simulink model "control2_feedback_linearization"  (R2023b)
settings: Solver=VariableStepAuto  StartTime=0.0  StopTime=20  RelTol=1e-3
values from neighbouring files (symbols this model uses):
  d = obs_r+threshold    (= 0.3)    [main.m]
  initial_position = [0,r]    [main.m]
  obs_r = 0.1    [main.m]
  obs_x = [20]    [main.m]
  obs_y = [20]    [main.m]
  parking_position = [0,0]    [main.m]
  r = 1    [main.m]
  T = 2*pi    (= 6.28318530718)    [main.m]
  t_values = 0:dt:T*1.1    [main.m]
  threshold = 0.2    [main.m]
undefined symbols (not defined in the file or in its folder): params
(part 1 of 3)
settings Model: Creator=djord  LastModifiedBy=djord

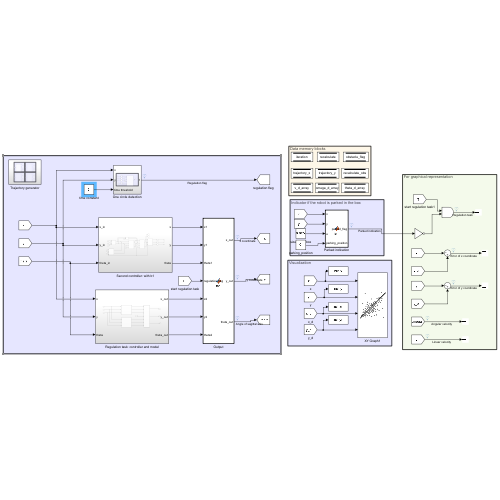
[thumbnail: Simulink's stored preview of the top-level diagram]
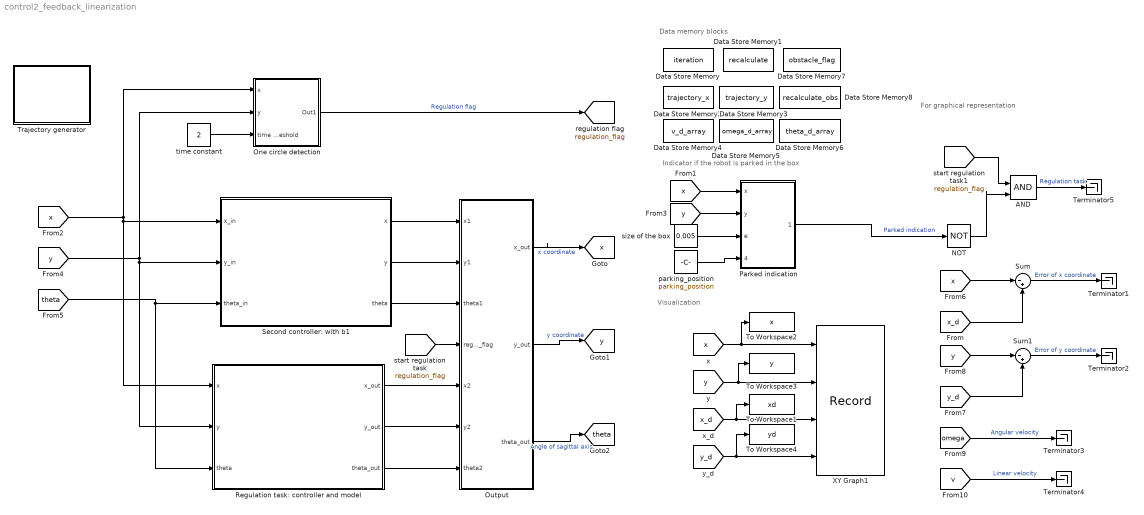
== system control2_feedback_linearization ==
  note: Indicator if the robot is parked in the box
  note: Visualization
  note: Data memory blocks
  note: For graphical representation
  AND : Logic  IconShape=distinctive  AllPortsSameDT=off  OutDataTypeStr=boolean
  Data Store Memory : DataStoreMemory  DataStoreName=iteration  WriteAfterWriteMsg=warning  ShowAdditionalParam=off
  Data Store Memory1 : DataStoreMemory  DataStoreName=recalculate  WriteAfterWriteMsg=warning  InitialValue=1  ShowAdditionalParam=off
  Data Store Memory2 : DataStoreMemory  DataStoreName=trajectory_x  WriteAfterWriteMsg=warning  InitialValue=zeros(length(t_values),1)  ShowAdditionalParam=off
  Data Store Memory3 : DataStoreMemory  DataStoreName=trajectory_y  WriteAfterWriteMsg=warning  InitialValue=zeros(length(t_values),1)  ShowAdditionalParam=off
  Data Store Memory4 : DataStoreMemory  DataStoreName=v_d_array  WriteAfterWriteMsg=warning  InitialValue=zeros(length(t_values),1)  ShowAdditionalParam=off
  Data Store Memory5 : DataStoreMemory  DataStoreName=omega_d_array  WriteAfterWriteMsg=warning  InitialValue=zeros(length(t_values),1)  ShowAdditionalParam=off
  Data Store Memory6 : DataStoreMemory  DataStoreName=theta_d_array  WriteAfterWriteMsg=warning  InitialValue=zeros(length(t_values),1)  ShowAdditionalParam=off
  Data Store Memory7 : DataStoreMemory  DataStoreName=obstacle_flag  ShowAdditionalParam=off
  Data Store Memory8 : DataStoreMemory  DataStoreName=recalculate_obs  WriteAfterWriteMsg=warning  ShowAdditionalParam=off
  NOT : Logic  Operator=NOT  IconShape=distinctive  AllPortsSameDT=off  OutDataTypeStr=boolean
  One circle detection : Subsystem
  Output : MATLAB Function  TreatAsAtomicUnit=on
  Parked indication : MATLAB Function  TreatAsAtomicUnit=on
  "Regulation task: controller and model " : Subsystem
  Second controller: with b1 : Subsystem
  Sum : Sum  Inputs=|-+
  Sum1 : Sum  Inputs=|-+
  Terminator{1..5} (5 alike) : Terminator
  To Workspace1 : ToWorkspace  VariableName=xd  SaveFormat=Timeseries  SampleTime=-1
  To Workspace2 : ToWorkspace  VariableName=x  SaveFormat=Timeseries  SampleTime=-1
  To Workspace3 : ToWorkspace  VariableName=y  SaveFormat=Timeseries  SampleTime=-1
  To Workspace4 : ToWorkspace  VariableName=yd  SaveFormat=Timeseries  SampleTime=-1
  Trajectory generator : Subsystem
  XY Graph1 : Record  FileSettingsInternal="{\"entries\":[{\"content\":{\"excelSettings\":{\"content\":{},\"type\":\"Streamout.ExcelSettings\"}},\"type\":\"Streamout.FileSettingStorage\",\"uuid\":\"\"}],\"packageUris\":[\"http:\\/\\/schema.mathworks.com\\/mf0\\/streamout_blocks\\/R2020a\"],\"version\":\"1.0\"}"  Layout=[1 1]  SignalsInternal="{\"entries\":[{\"content\":{\"signals\":[{\"content\":{\"blockPath\":[],\"dimensions\":[1],\"domain\":\"\",\"lineColor\":\"#139fff\",\"port\":1,\"sid\":[\"\"],\"signalID\":1,\"signalName\":\"x\"},\"type\":\"RecordBlkView.Signal\",\"uuid\":\"\"},{\"content\":{\"blockPath\":[],\"dimensions\":[1],\"domain\":\"\",\"lineColor\":\"#ff6929\",\"port\":2,\"sid\":[\"\"],\"signalID\":2,\"signalName\":\"y\"},\"type\":\"RecordBlkView.Signal\",\"uuid\":\"\"},{\"content\":{\"blockPath\":[],\"dimensions\":[1],\"domain\":\"\",\"lineColor\":\"#b746ff\",\"port\":3,\"sid\":[\"\"],\"signalID\":3,\"signalName\":\"x_d\"},\"type\":\"RecordBlkView.Signal\",\"uuid\":\"\"},{\"content\":{\"blockPath\":[],\"dimensions\":[1],\"domain\":\"\",\"lineColor\":\"#64d413\",\"port\":4,\"sid\":[\"\"],\"signalID\":4,\"signalName\":\"y_d\"},\"type\":\"RecordBlkView.Signal\",\"uuid\":\"\"}]},\"type\":\"RecordBlkView.InputSignals\",\"uuid\":\"\"}],\"packageUris\":[\"http:\\/\\/schema.mathworks.com\\/mf0\\/streamout_blocks\\/R2020a\"],\"version\":\"1.0\"}"  VisualizationBindings="{\"xyplotplugin\":{\"info\":[{\"series\":[],\"subplotID\":1}]}}"  CompatibilityTag=XY  st=-1
  parking_position : Constant  Value=parking_position
  size of the box : Constant  Value=0.005
  time constant : Constant  Value=2
  tag scope: regulation_flag=global, theta=global, x=global, y=global
  wires:
  [x] -> To Workspace2/1, XY Graph1/1
  [y] -> To Workspace3/1, XY Graph1/2
  [x_d] -> XY Graph1/3, To Workspace1/1
  [y_d] -> To Workspace4/1, XY Graph1/4
  "Regulation task: controller and model "/1(x_out) -> Output/5(x2)
  "Regulation task: controller and model "/2(y_out) -> Output/6(y2)
  "Regulation task: controller and model "/3(theta_out) -> Output/7(theta2)
  [regulation_flag] -> Output/4(regulation_flag)
  One circle detection/1(Out1) -> [regulation_flag]  "Regulation flag"
  time constant/1 -> One circle detection/3(time threshold)
  Output/1(x_out) -> [x]  "x coordinate"
  Output/2(y_out) -> [y]  "y coordinate"
  Output/3(theta_out) -> [theta]  "Angle of sagittal axis"
  [x] -> Parked indication/1(x)
  [y] -> Parked indication/2(y)
  size of the box/1 -> Parked indication/3(e)
  Second controller: with b1/1(x) -> Output/1(x1)
  Second controller: with b1/2(y) -> Output/2(y1)
  Second controller: with b1/3(theta) -> Output/3(theta1)
  [x] -> "Regulation task: controller and model "/1(x), Second controller: with b1/1(x_in), One circle detection/1(x)
  [y] -> "Regulation task: controller and model "/2(y), Second controller: with b1/2(y_in), One circle detection/2(y)
  [theta] -> "Regulation task: controller and model "/3(theta), Second controller: with b1/3(theta_in)
  AND/1 -> Terminator5/1  "Regulation task"
  [x_d] -> Sum/2
  [regulation_flag] -> AND/1
  [v] -> Terminator4/1  "Linear velocity"
  [x] -> Sum/1
  [y_d] -> Sum1/2
  [y] -> Sum1/1
  NOT/1 -> AND/2
  [omega] -> Terminator3/1  "Angular velocity"
  Parked indication/1(parked_flag) -> NOT/1  "Parked indication"
  Sum/1 -> Terminator1/1  "Error of x coordinate"
  Sum1/1 -> Terminator2/1  "Error of y coordinate"
  parking_position/1 -> Parked indication/4(parking_position)

== system control2_feedback_linearization/One circle detection ==
  note: One circle detection: unit delay needed to avoid algebraic loop
  x : Inport
  y : Inport  Port=2
  time threshold : Inport  Port=3
  Clock : Clock
  Unit Delay{1..4} (4 alike) : UnitDelay  SampleTime=-1  HasFrameUpgradeWarning=on
  initial position1 : Constant  Value=initial_position
  one circle detection : MATLAB Function  TreatAsAtomicUnit=on
  Out1 : Outport
  wires:
  one circle detection/1(regulation_flag) -> Out1/1
  initial position1/1 -> one circle detection/4(initial_position)
  Clock/1 -> Unit Delay2/1
  Unit Delay2/1 -> one circle detection/1(t)
  [regulation_flag] -> Unit Delay3/1
  Unit Delay3/1 -> one circle detection/5(regulation_flag_previous)
  time threshold/1 -> one circle detection/6(constant)
  x/1 -> Unit Delay1/1
  y/1 -> Unit Delay4/1
  Unit Delay1/1 -> one circle detection/2(x)
  Unit Delay4/1 -> one circle detection/3(y)

== system control2_feedback_linearization/Regulation task: controller and model  ==
  x : Inport
  y : Inport  Port=2
  theta : Inport  Port=3
  Cartesian Controller : Subsystem
  Choice of regulation controller : Constant
  Controller with polar coordinates : Subsystem
  Regulation controller choice : MATLAB Function  TreatAsAtomicUnit=on
  x_out : Outport
  y_out : Outport  Port=2
  theta_out : Outport  Port=3
  wires:
  y/1 -> Cartesian Controller/2(y), Controller with polar coordinates/2(y)
  theta/1 -> Cartesian Controller/3(theta), Controller with polar coordinates/3(theta)
  Regulation controller choice/1(x_out) -> x_out/1
  Regulation controller choice/3(theta_out) -> theta_out/1
  Regulation controller choice/2(y_out) -> y_out/1
  Choice of regulation controller/1 -> Regulation controller choice/4(controller_choice)
  Cartesian Controller/1(x1) -> Regulation controller choice/1(x1)
  Cartesian Controller/2(y1) -> Regulation controller choice/2(y1)
  Cartesian Controller/3(theta1) -> Regulation controller choice/3(theta1)
  Controller with polar coordinates/1(x_out) -> Regulation controller choice/5(x2)
  Controller with polar coordinates/2(y_out) -> Regulation controller choice/6(y2)
  Controller with polar coordinates/3(theta_out) -> Regulation controller choice/7(theta2)
  x/1 -> Cartesian Controller/1(x), Controller with polar coordinates/1(x)

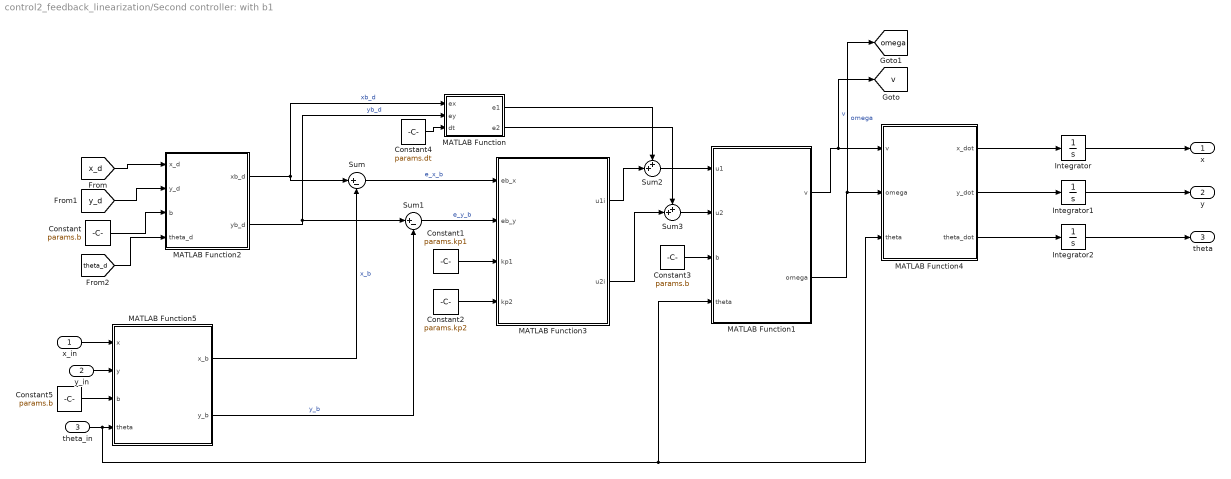
== system control2_feedback_linearization/Second controller: with b1 ==
  x_in : Inport
  y_in : Inport  Port=2
  theta_in : Inport  Port=3
  Constant : Constant  Value=params.b
  Constant1 : Constant  Value=params.kp1
  Constant2 : Constant  Value=params.kp2
  Constant3 : Constant  Value=params.b
  Constant4 : Constant  Value=params.dt
  Constant5 : Constant  Value=params.b
  Integrator : Integrator
  Integrator1 : Integrator  InitialCondition=1
  Integrator2 : Integrator
  MATLAB Function : MATLAB Function  TreatAsAtomicUnit=on
  MATLAB Function1 : MATLAB Function  TreatAsAtomicUnit=on
  MATLAB Function2 : MATLAB Function  TreatAsAtomicUnit=on
  MATLAB Function3 : MATLAB Function  TreatAsAtomicUnit=on
  MATLAB Function4 : MATLAB Function  TreatAsAtomicUnit=on
  MATLAB Function5 : MATLAB Function  TreatAsAtomicUnit=on
  Sum : Sum  Inputs=|+-
  Sum1 : Sum  Inputs=|+-
  Sum2 : Sum  Inputs=++|
  Sum3 : Sum  Inputs=++|
  x : Outport
  y : Outport  Port=2
  theta : Outport  Port=3
  tag scope: omega=global, v=global
  wires:
  MATLAB Function4/3(theta_dot) -> Integrator2/1
  MATLAB Function1/2(omega) -> [omega], MATLAB Function4/2(omega)  "omega"
  Sum3/1 -> MATLAB Function1/2(u2)
  MATLAB Function1/1(v) -> [v], MATLAB Function4/1(v)  "v"
  Constant1/1 -> MATLAB Function3/3(kp1)
  MATLAB Function3/1(u1i) -> Sum2/2
  Constant/1 -> MATLAB Function2/3(b)
  Constant2/1 -> MATLAB Function3/4(kp2)
  MATLAB Function5/2(y_b) -> Sum1/2  "y_b"
  Sum2/1 -> MATLAB Function1/1(u1)
  Integrator2/1 -> theta/1
  MATLAB Function5/1(x_b) -> Sum/2  "x_b"
  Integrator1/1 -> y/1
  Constant3/1 -> MATLAB Function1/3(b)
  Sum1/1 -> MATLAB Function3/2(eb_y)  "e_y_b"
  MATLAB Function4/1(x_dot) -> Integrator/1
  MATLAB Function3/2(u2i) -> Sum3/2
  Sum/1 -> MATLAB Function3/1(eb_x)  "e_x_b"
  MATLAB Function2/2(yb_d) -> MATLAB Function/2(ey), Sum1/1  "yb_d"
  Integrator/1 -> x/1
  MATLAB Function4/2(y_dot) -> Integrator1/1
  MATLAB Function2/1(xb_d) -> MATLAB Function/1(ex), Sum/1  "xb_d"
  Constant5/1 -> MATLAB Function5/3(b)
  [x_d] -> MATLAB Function2/1(x_d)
  [y_d] -> MATLAB Function2/2(y_d)
  [theta_d] -> MATLAB Function2/4(theta_d)
  MATLAB Function/1(e1) -> Sum2/1
  MATLAB Function/2(e2) -> Sum3/1
  Constant4/1 -> MATLAB Function/3(dt)
  x_in/1 -> MATLAB Function5/1(x)
  y_in/1 -> MATLAB Function5/2(y)
  theta_in/1 -> MATLAB Function1/4(theta), MATLAB Function4/3(theta), MATLAB Function5/4(theta)

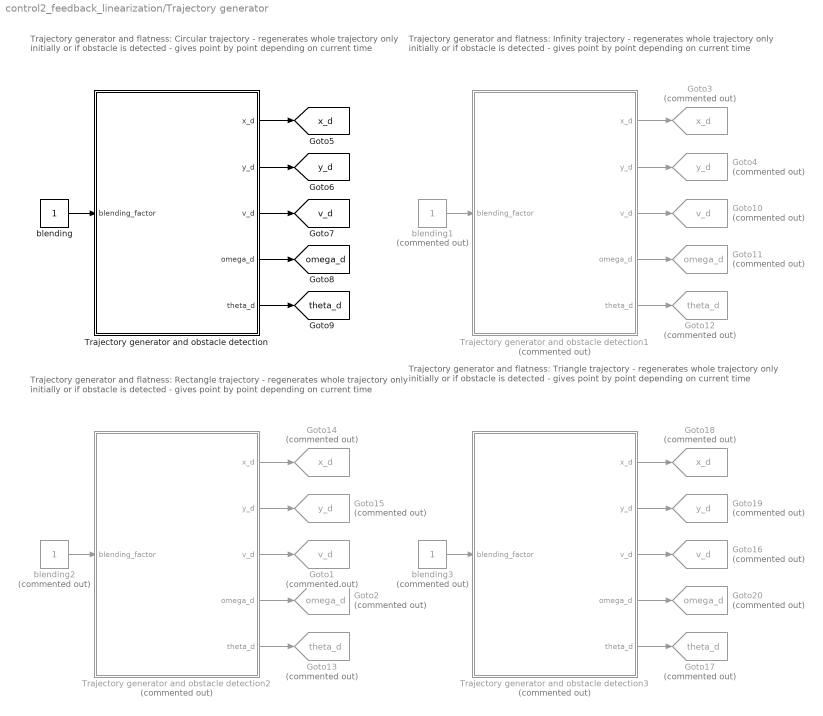
== system control2_feedback_linearization/Trajectory generator ==
  note: Trajectory generator and flatness: Infinity trajectory
      |
      | - regenerates whole trajectory only initially or if obstacle is detected
      | - gives point by point depending on current time
  note: Trajectory generator and flatness: Circular trajectory
      |
      | - regenerates whole trajectory only initially or if obstacle is detected
      | - gives point by point depending on current time
  note: Trajectory generator and flatness: Rectangle trajectory
      |
      | - regenerates whole trajectory only initially or if obstacle is detected
      | - gives point by point depending on current time
  note: Trajectory generator and flatness: Triangle trajectory
      |
      | - regenerates whole trajectory only initially or if obstacle is detected
      | - gives point by point depending on current time
  Goto1 : Goto  Commented=on  GotoTag=v_d  TagVisibility=global
  Goto10 : Goto  Commented=on  GotoTag=v_d  TagVisibility=global
  Goto11 : Goto  Commented=on  GotoTag=omega_d  TagVisibility=global
  Goto12 : Goto  Commented=on  GotoTag=theta_d  TagVisibility=global
  Goto13 : Goto  Commented=on  GotoTag=theta_d  TagVisibility=global
  Goto14 : Goto  Commented=on  GotoTag=x_d  TagVisibility=global
  Goto15 : Goto  Commented=on  GotoTag=y_d  TagVisibility=global
  Goto16 : Goto  Commented=on  GotoTag=v_d  TagVisibility=global
  Goto17 : Goto  Commented=on  GotoTag=theta_d  TagVisibility=global
  Goto18 : Goto  Commented=on  GotoTag=x_d  TagVisibility=global
  Goto19 : Goto  Commented=on  GotoTag=y_d  TagVisibility=global
  Goto2 : Goto  Commented=on  GotoTag=omega_d  TagVisibility=global
  Goto20 : Goto  Commented=on  GotoTag=omega_d  TagVisibility=global
  Goto3 : Goto  Commented=on  GotoTag=x_d  TagVisibility=global
  Goto4 : Goto  Commented=on  GotoTag=y_d  TagVisibility=global
  Trajectory generator and obstacle detection : Subsystem
  Trajectory generator and obstacle detection1 : Subsystem  Commented=on
  Trajectory generator and obstacle detection2 : Subsystem  Commented=on
  Trajectory generator and obstacle detection3 : Subsystem  Commented=on
  blending : Constant
  blending1 : Constant  Commented=on
  blending2 : Constant  Commented=on
  blending3 : Constant  Commented=on
  tag scope: omega_d=global, theta_d=global, v_d=global, x_d=global, y_d=global
  wires:
  blending1/1 -> Trajectory generator and obstacle detection1/1(blending_factor)
  Trajectory generator and obstacle detection/5(theta_d) -> [theta_d]
  Trajectory generator and obstacle detection1/3(v_d) -> Goto10/1
  Trajectory generator and obstacle detection1/2(y_d) -> Goto4/1
  Trajectory generator and obstacle detection1/1(x_d) -> Goto3/1
  Trajectory generator and obstacle detection/2(y_d) -> [y_d]
  Trajectory generator and obstacle detection1/4(omega_d) -> Goto11/1
  Trajectory generator and obstacle detection/3(v_d) -> [v_d]
  Trajectory generator and obstacle detection/4(omega_d) -> [omega_d]
  Trajectory generator and obstacle detection/1(x_d) -> [x_d]
  Trajectory generator and obstacle detection1/5(theta_d) -> Goto12/1
  blending/1 -> Trajectory generator and obstacle detection/1(blending_factor)
  blending2/1 -> Trajectory generator and obstacle detection2/1(blending_factor)
  Trajectory generator and obstacle detection2/4(omega_d) -> Goto2/1
  Trajectory generator and obstacle detection2/3(v_d) -> Goto1/1
  Trajectory generator and obstacle detection2/2(y_d) -> Goto15/1
  Trajectory generator and obstacle detection2/5(theta_d) -> Goto13/1
  Trajectory generator and obstacle detection2/1(x_d) -> Goto14/1
  Trajectory generator and obstacle detection3/2(y_d) -> Goto19/1
  Trajectory generator and obstacle detection3/4(omega_d) -> Goto20/1
  blending3/1 -> Trajectory generator and obstacle detection3/1(blending_factor)
  Trajectory generator and obstacle detection3/5(theta_d) -> Goto17/1
  Trajectory generator and obstacle detection3/3(v_d) -> Goto16/1
  Trajectory generator and obstacle detection3/1(x_d) -> Goto18/1

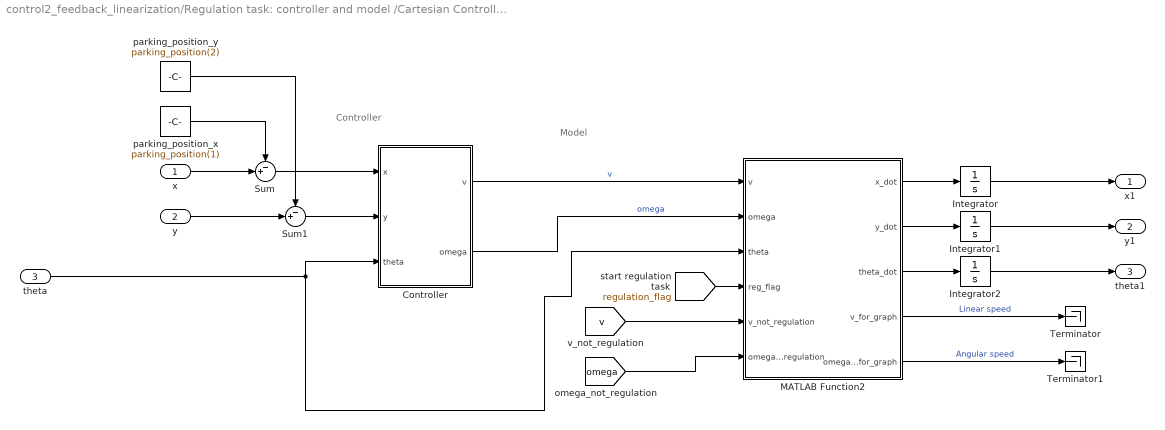
== system control2_feedback_linearization/Regulation task: controller and model /Cartesian Controller ==
  note: Model
  note: Controller
  x : Inport
  y : Inport  Port=2
  theta : Inport  Port=3
  Controller : MATLAB Function  TreatAsAtomicUnit=on
  Integrator : Integrator
  Integrator1 : Integrator  InitialCondition=1
  Integrator2 : Integrator
  MATLAB Function2 : MATLAB Function  TreatAsAtomicUnit=on
  Sum : Sum  Inputs=-+|
  Sum1 : Sum  Inputs=-+|
  Terminator : Terminator
  Terminator1 : Terminator
  parking_position_x : Constant  Value=parking_position(1)
  parking_position_y : Constant  Value=parking_position(2)
  x1 : Outport
  y1 : Outport  Port=2
  theta1 : Outport  Port=3
  wires:
  MATLAB Function2/1(x_dot) -> Integrator/1
  Controller/1(v) -> MATLAB Function2/1(v)  "v"
  [regulation_flag] -> MATLAB Function2/4(reg_flag)
  Controller/2(omega) -> MATLAB Function2/2(omega)  "omega"
  MATLAB Function2/3(theta_dot) -> Integrator2/1
  MATLAB Function2/2(y_dot) -> Integrator1/1
  Integrator/1 -> x1/1
  Integrator1/1 -> y1/1
  x/1 -> Sum/2
  parking_position_x/1 -> Sum/1
  Sum/1 -> Controller/1(x)
  y/1 -> Sum1/2
  Sum1/1 -> Controller/2(y)
  parking_position_y/1 -> Sum1/1
  [v] -> MATLAB Function2/5(v_not_regulation)
  [omega] -> MATLAB Function2/6(omega_not_regulation)
  MATLAB Function2/4(v_for_graph) -> Terminator/1  "Linear speed"
  MATLAB Function2/5(omega_for_graph) -> Terminator1/1  "Angular speed"
  theta/1 -> MATLAB Function2/3(theta), Controller/3(theta)
  Integrator2/1 -> theta1/1

== system control2_feedback_linearization/Regulation task: controller and model /Controller with polar coordinates ==
  note: Model
  note: Controller
  x : Inport
  y : Inport  Port=2
  theta : Inport  Port=3
  Controller : MATLAB Function  TreatAsAtomicUnit=on
  Integrator : Integrator
  Integrator1 : Integrator
  Integrator2 : Integrator
  Saturation : Saturate
  Saturation1 : Saturate  UpperLimit=2  LowerLimit=-2
  Transformation to Cartesian coordinates : MATLAB Function  TreatAsAtomicUnit=on
  Transformation to polar coordinates : MATLAB Function  TreatAsAtomicUnit=on
  Unicycle model: polar coordinates : MATLAB Function  TreatAsAtomicUnit=on
  x_out : Outport
  y_out : Outport  Port=2
  theta_out : Outport  Port=3
  wires:
  Transformation to polar coordinates/3(delta) -> Controller/2(delta)
  Integrator2/1 -> Transformation to Cartesian coordinates/3(delta)
  Unicycle model: polar coordinates/2(gamma_dot) -> Integrator1/1
  Unicycle model: polar coordinates/1(rho_dot) -> Integrator/1
  Integrator/1 -> Transformation to Cartesian coordinates/1(rho)
  Unicycle model: polar coordinates/3(delta_dot) -> Integrator2/1
  Integrator1/1 -> Transformation to Cartesian coordinates/2(gamma)
  Transformation to Cartesian coordinates/1(x) -> x_out/1
  Transformation to Cartesian coordinates/2(y) -> y_out/1
  Transformation to Cartesian coordinates/3(theta) -> theta_out/1
  x/1 -> Transformation to polar coordinates/1(x)
  y/1 -> Transformation to polar coordinates/2(y)
  theta/1 -> Transformation to polar coordinates/3(theta)
  Controller/2(omega) -> Saturation1/1
  Transformation to polar coordinates/2(gamma) -> Unicycle model: polar coordinates/2(gamma), Controller/1(gamma)
  Transformation to polar coordinates/1(rho) -> Unicycle model: polar coordinates/1(rho)
  [regulation_flag] -> Unicycle model: polar coordinates/5(regulation_flag)
  Saturation/1 -> Unicycle model: polar coordinates/3(u)
  Saturation1/1 -> Unicycle model: polar coordinates/4(omega)
  Controller/1(u) -> Saturation/1

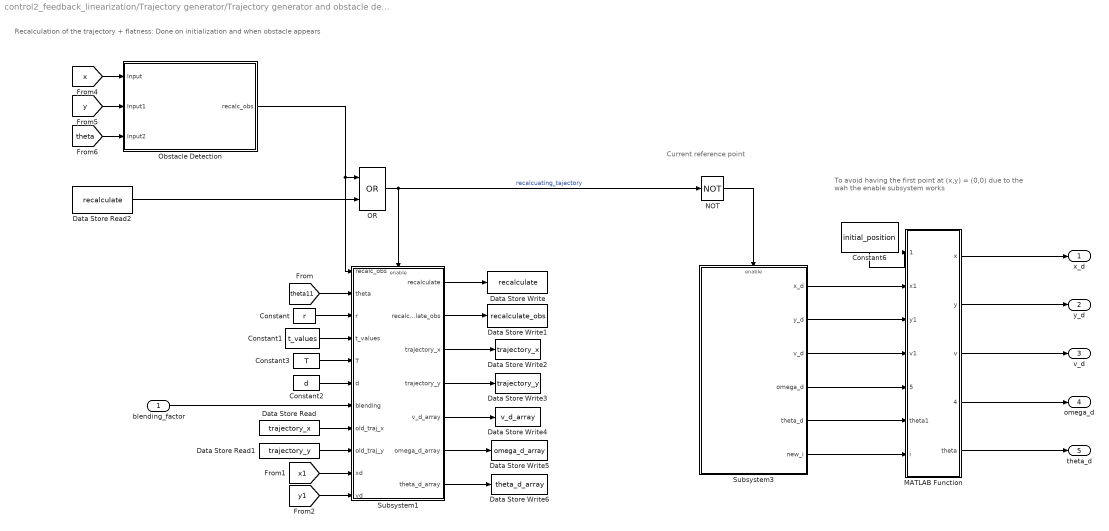
== system control2_feedback_linearization/Trajectory generator/Trajectory generator and obstacle detection ==
  note: To avoid having the first point at (x,y) = (0,0)
      | due to the wah the enable subsystem works
  note: Recalculation of the trajectory + flatness:
      | Done on initialization and when obstacle appears
  note: Current reference point
  blending_factor : Inport
  Constant : Constant  Value=r
  Constant1 : Constant  Value=t_values
  Constant2 : Constant  Value=d
  Constant3 : Constant  Value=T
  Constant6 : Constant  Value=initial_position
  Data Store Read : DataStoreRead  DataStoreName=trajectory_x  IndexOptions=Index vector (dialog)  Indices=1  OutputSizes=1
  Data Store Read1 : DataStoreRead  DataStoreName=trajectory_y  IndexOptions=Index vector (dialog)  Indices=1  OutputSizes=1
  Data Store Read2 : DataStoreRead  DataStoreName=recalculate  IndexOptions=Index vector (dialog)  Indices=1  OutputSizes=1
  Data Store Write : DataStoreWrite  DataStoreName=recalculate  IndexOptions=Index vector (dialog)  Indices=1  OutputSizes=1
  Data Store Write1 : DataStoreWrite  DataStoreName=recalculate_obs  IndexOptions=Index vector (dialog)  Indices=1  OutputSizes=1
  Data Store Write2 : DataStoreWrite  DataStoreName=trajectory_x  IndexOptions=Index vector (dialog)  Indices=1  OutputSizes=1
  Data Store Write3 : DataStoreWrite  DataStoreName=trajectory_y  IndexOptions=Index vector (dialog)  Indices=1  OutputSizes=1
  Data Store Write4 : DataStoreWrite  DataStoreName=v_d_array  IndexOptions=Index vector (dialog)  Indices=1  OutputSizes=1
  Data Store Write5 : DataStoreWrite  DataStoreName=omega_d_array  IndexOptions=Index vector (dialog)  Indices=1  OutputSizes=1
  Data Store Write6 : DataStoreWrite  DataStoreName=theta_d_array  IndexOptions=Index vector (dialog)  Indices=1  OutputSizes=1
  MATLAB Function : MATLAB Function  TreatAsAtomicUnit=on
  NOT : Logic  Operator=NOT  IconShape=distinctive  AllPortsSameDT=off  OutDataTypeStr=boolean
  OR : Logic  Operator=OR  IconShape=distinctive  AllPortsSameDT=off  OutDataTypeStr=boolean
  Obstacle Detection : Subsystem
  Subsystem1 : Subsystem
  Subsystem3 : Subsystem
  x_d : Outport
  y_d : Outport  Port=2
  v_d : Outport  Port=3
  omega_d : Outport  Port=4
  theta_d : Outport  Port=5
  wires:
  Constant/1 -> Subsystem1/3(r)
  Constant1/1 -> Subsystem1/4(t_values)
  NOT/1 -> Subsystem3/Enable
  Constant2/1 -> Subsystem1/6(d)
  Data Store Read2/1 -> OR/2
  OR/1 -> NOT/1, Subsystem1/Enable  "recalcuating_tajectory"
  Subsystem1/7(theta_d_array) -> Data Store Write6/1
  Subsystem1/6(omega_d_array) -> Data Store Write5/1
  Subsystem1/5(v_d_array) -> Data Store Write4/1
  Subsystem1/4(trajectory_y) -> Data Store Write3/1
  Subsystem1/3(trajectory_x) -> Data Store Write2/1
  Subsystem1/1(recalculate) -> Data Store Write/1
  Constant3/1 -> Subsystem1/5(T)
  Subsystem3/1(x_d) -> MATLAB Function/2(x1)
  MATLAB Function/1(x) -> x_d/1
  Subsystem3/2(y_d) -> MATLAB Function/3(y1)
  MATLAB Function/2(y) -> y_d/1
  MATLAB Function/3(v) -> v_d/1
  Subsystem3/3(v_d) -> MATLAB Function/4(v1)
  Subsystem3/4(omega_d) -> MATLAB Function/5(omega1)
  Subsystem3/5(theta_d) -> MATLAB Function/6(theta1)
  MATLAB Function/4(omega) -> omega_d/1
  MATLAB Function/5(theta) -> theta_d/1
  Constant6/1 -> MATLAB Function/1(initial_position)
  Subsystem3/6(new_i) -> MATLAB Function/7(i)
  Subsystem1/2(recalculate_obs) -> Data Store Write1/1
  blending_factor/1 -> Subsystem1/7(blending)
  Data Store Read/1 -> Subsystem1/8(old_traj_x)
  Data Store Read1/1 -> Subsystem1/9(old_traj_y)
  [x1] -> Subsystem1/10(xd)
  [y1] -> Subsystem1/11(yd)
  [theta11] -> Subsystem1/2(theta)
  [x] -> Obstacle Detection/1(Input)
  Obstacle Detection/1(recalc_obs) -> OR/1, Subsystem1/1(recalc_obs)
  [theta] -> Obstacle Detection/3(Input2)
  [y] -> Obstacle Detection/2(Input1)

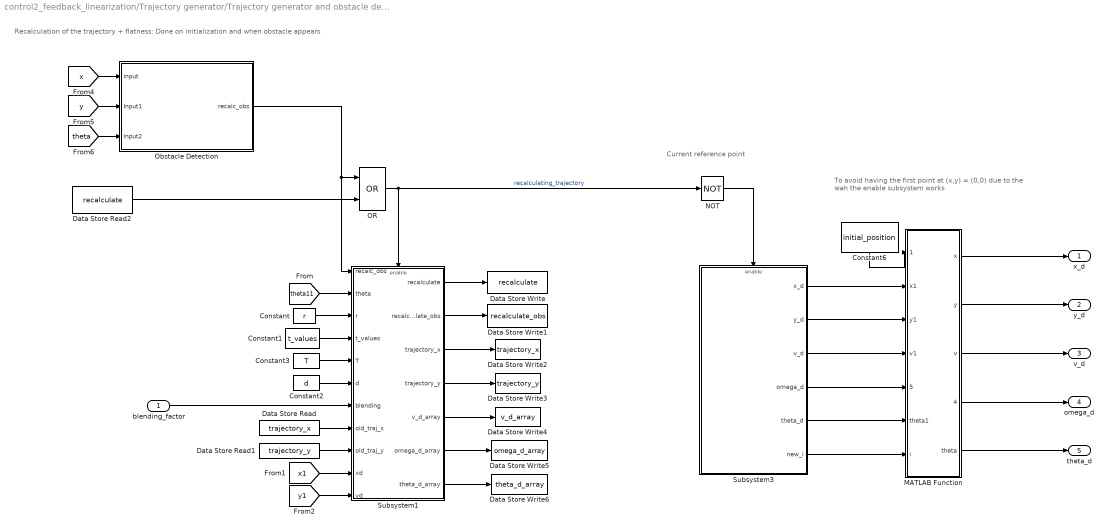
== system control2_feedback_linearization/Trajectory generator/Trajectory generator and obstacle detection1 ==
  note: To avoid having the first point at (x,y) = (0,0)
      | due to the wah the enable subsystem works
  note: Recalculation of the trajectory + flatness:
      | Done on initialization and when obstacle appears
  note: Current reference point
  blending_factor : Inport
  Constant : Constant  Value=r
  Constant1 : Constant  Value=t_values
  Constant2 : Constant  Value=d
  Constant3 : Constant  Value=T
  Constant6 : Constant  Value=initial_position
  Data Store Read : DataStoreRead  DataStoreName=trajectory_x  IndexOptions=Index vector (dialog)  Indices=1  OutputSizes=1
  Data Store Read1 : DataStoreRead  DataStoreName=trajectory_y  IndexOptions=Index vector (dialog)  Indices=1  OutputSizes=1
  Data Store Read2 : DataStoreRead  DataStoreName=recalculate  IndexOptions=Index vector (dialog)  Indices=1  OutputSizes=1
  Data Store Write : DataStoreWrite  DataStoreName=recalculate  IndexOptions=Index vector (dialog)  Indices=1  OutputSizes=1
  Data Store Write1 : DataStoreWrite  DataStoreName=recalculate_obs  IndexOptions=Index vector (dialog)  Indices=1  OutputSizes=1
  Data Store Write2 : DataStoreWrite  DataStoreName=trajectory_x  IndexOptions=Index vector (dialog)  Indices=1  OutputSizes=1
  Data Store Write3 : DataStoreWrite  DataStoreName=trajectory_y  IndexOptions=Index vector (dialog)  Indices=1  OutputSizes=1
  Data Store Write4 : DataStoreWrite  DataStoreName=v_d_array  IndexOptions=Index vector (dialog)  Indices=1  OutputSizes=1
  Data Store Write5 : DataStoreWrite  DataStoreName=omega_d_array  IndexOptions=Index vector (dialog)  Indices=1  OutputSizes=1
  Data Store Write6 : DataStoreWrite  DataStoreName=theta_d_array  IndexOptions=Index vector (dialog)  Indices=1  OutputSizes=1
  MATLAB Function : MATLAB Function  TreatAsAtomicUnit=on
  NOT : Logic  Operator=NOT  IconShape=distinctive  AllPortsSameDT=off  OutDataTypeStr=boolean
  OR : Logic  Operator=OR  IconShape=distinctive  AllPortsSameDT=off  OutDataTypeStr=boolean
  Obstacle Detection : Subsystem
  Subsystem1 : Subsystem
  Subsystem3 : Subsystem
  x_d : Outport
  y_d : Outport  Port=2
  v_d : Outport  Port=3
  omega_d : Outport  Port=4
  theta_d : Outport  Port=5
  wires:
  Constant/1 -> Subsystem1/3(r)
  Constant1/1 -> Subsystem1/4(t_values)
  NOT/1 -> Subsystem3/Enable
  Constant2/1 -> Subsystem1/6(d)
  Data Store Read2/1 -> OR/2
  OR/1 -> NOT/1, Subsystem1/Enable  "recalculating_trajectory"
  Subsystem1/7(theta_d_array) -> Data Store Write6/1
  Subsystem1/6(omega_d_array) -> Data Store Write5/1
  Subsystem1/5(v_d_array) -> Data Store Write4/1
  Subsystem1/4(trajectory_y) -> Data Store Write3/1
  Subsystem1/3(trajectory_x) -> Data Store Write2/1
  Subsystem1/1(recalculate) -> Data Store Write/1
  Constant3/1 -> Subsystem1/5(T)
  Subsystem3/1(x_d) -> MATLAB Function/2(x1)
  MATLAB Function/1(x) -> x_d/1
  Subsystem3/2(y_d) -> MATLAB Function/3(y1)
  MATLAB Function/2(y) -> y_d/1
  MATLAB Function/3(v) -> v_d/1
  Subsystem3/3(v_d) -> MATLAB Function/4(v1)
  Subsystem3/4(omega_d) -> MATLAB Function/5(omega1)
  Subsystem3/5(theta_d) -> MATLAB Function/6(theta1)
  MATLAB Function/4(omega) -> omega_d/1
  MATLAB Function/5(theta) -> theta_d/1
  Constant6/1 -> MATLAB Function/1(initial_position)
  Subsystem3/6(new_i) -> MATLAB Function/7(i)
  Subsystem1/2(recalculate_obs) -> Data Store Write1/1
  blending_factor/1 -> Subsystem1/7(blending)
  Data Store Read/1 -> Subsystem1/8(old_traj_x)
  Data Store Read1/1 -> Subsystem1/9(old_traj_y)
  Obstacle Detection/1(recalc_obs) -> Subsystem1/1(recalc_obs), OR/1
  [x] -> Obstacle Detection/1(Input)
  [y] -> Obstacle Detection/2(Input1)
  [theta] -> Obstacle Detection/3(Input2)
  [x1] -> Subsystem1/10(xd)
  [y1] -> Subsystem1/11(yd)
  [theta11] -> Subsystem1/2(theta)

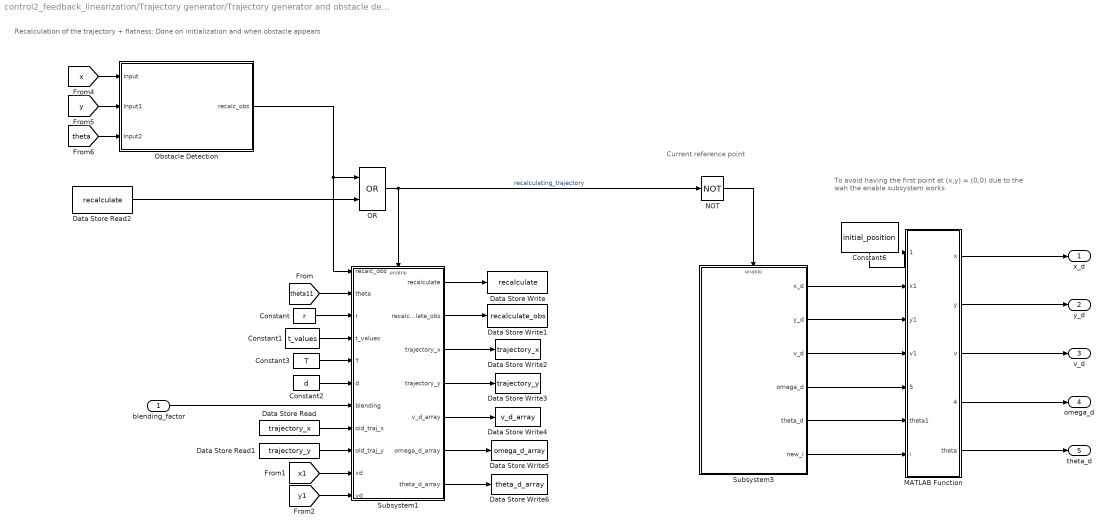
== system control2_feedback_linearization/Trajectory generator/Trajectory generator and obstacle detection2 ==
  note: To avoid having the first point at (x,y) = (0,0)
      | due to the wah the enable subsystem works
  note: Recalculation of the trajectory + flatness:
      | Done on initialization and when obstacle appears
  note: Current reference point
  blending_factor : Inport
  Constant : Constant  Value=r
  Constant1 : Constant  Value=t_values
  Constant2 : Constant  Value=d
  Constant3 : Constant  Value=T
  Constant6 : Constant  Value=initial_position
  Data Store Read : DataStoreRead  DataStoreName=trajectory_x  IndexOptions=Index vector (dialog)  Indices=1  OutputSizes=1
  Data Store Read1 : DataStoreRead  DataStoreName=trajectory_y  IndexOptions=Index vector (dialog)  Indices=1  OutputSizes=1
  Data Store Read2 : DataStoreRead  DataStoreName=recalculate  IndexOptions=Index vector (dialog)  Indices=1  OutputSizes=1
  Data Store Write : DataStoreWrite  DataStoreName=recalculate  IndexOptions=Index vector (dialog)  Indices=1  OutputSizes=1
  Data Store Write1 : DataStoreWrite  DataStoreName=recalculate_obs  IndexOptions=Index vector (dialog)  Indices=1  OutputSizes=1
  Data Store Write2 : DataStoreWrite  DataStoreName=trajectory_x  IndexOptions=Index vector (dialog)  Indices=1  OutputSizes=1
  Data Store Write3 : DataStoreWrite  DataStoreName=trajectory_y  IndexOptions=Index vector (dialog)  Indices=1  OutputSizes=1
  Data Store Write4 : DataStoreWrite  DataStoreName=v_d_array  IndexOptions=Index vector (dialog)  Indices=1  OutputSizes=1
  Data Store Write5 : DataStoreWrite  DataStoreName=omega_d_array  IndexOptions=Index vector (dialog)  Indices=1  OutputSizes=1
  Data Store Write6 : DataStoreWrite  DataStoreName=theta_d_array  IndexOptions=Index vector (dialog)  Indices=1  OutputSizes=1
  MATLAB Function : MATLAB Function  TreatAsAtomicUnit=on
  NOT : Logic  Operator=NOT  IconShape=distinctive  AllPortsSameDT=off  OutDataTypeStr=boolean
  OR : Logic  Operator=OR  IconShape=distinctive  AllPortsSameDT=off  OutDataTypeStr=boolean
  Obstacle Detection : Subsystem
  Subsystem1 : Subsystem
  Subsystem3 : Subsystem
  x_d : Outport
  y_d : Outport  Port=2
  v_d : Outport  Port=3
  omega_d : Outport  Port=4
  theta_d : Outport  Port=5
  wires:
  Constant/1 -> Subsystem1/3(r)
  Constant1/1 -> Subsystem1/4(t_values)
  NOT/1 -> Subsystem3/Enable
  Constant2/1 -> Subsystem1/6(d)
  Data Store Read2/1 -> OR/2
  OR/1 -> NOT/1, Subsystem1/Enable  "recalculating_trajectory"
  Subsystem1/7(theta_d_array) -> Data Store Write6/1
  Subsystem1/6(omega_d_array) -> Data Store Write5/1
  Subsystem1/5(v_d_array) -> Data Store Write4/1
  Subsystem1/4(trajectory_y) -> Data Store Write3/1
  Subsystem1/3(trajectory_x) -> Data Store Write2/1
  Subsystem1/1(recalculate) -> Data Store Write/1
  Constant3/1 -> Subsystem1/5(T)
  Subsystem3/1(x_d) -> MATLAB Function/2(x1)
  MATLAB Function/1(x) -> x_d/1
  Subsystem3/2(y_d) -> MATLAB Function/3(y1)
  MATLAB Function/2(y) -> y_d/1
  MATLAB Function/3(v) -> v_d/1
  Subsystem3/3(v_d) -> MATLAB Function/4(v1)
  Subsystem3/4(omega_d) -> MATLAB Function/5(omega1)
  Subsystem3/5(theta_d) -> MATLAB Function/6(theta1)
  MATLAB Function/4(omega) -> omega_d/1
  MATLAB Function/5(theta) -> theta_d/1
  Constant6/1 -> MATLAB Function/1(initial_position)
  Subsystem3/6(new_i) -> MATLAB Function/7(i)
  Subsystem1/2(recalculate_obs) -> Data Store Write1/1
  blending_factor/1 -> Subsystem1/7(blending)
  Data Store Read/1 -> Subsystem1/8(old_traj_x)
  Data Store Read1/1 -> Subsystem1/9(old_traj_y)
  Obstacle Detection/1(recalc_obs) -> OR/1, Subsystem1/1(recalc_obs)
  [x] -> Obstacle Detection/1(Input)
  [y] -> Obstacle Detection/2(Input1)
  [theta] -> Obstacle Detection/3(Input2)
  [x1] -> Subsystem1/10(xd)
  [y1] -> Subsystem1/11(yd)
  [theta11] -> Subsystem1/2(theta)

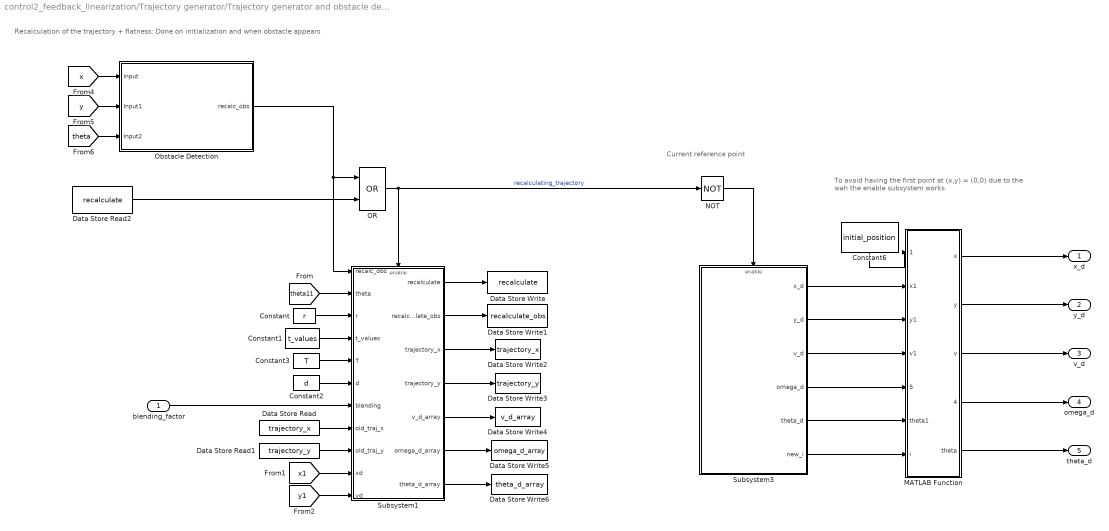
== system control2_feedback_linearization/Trajectory generator/Trajectory generator and obstacle detection3 ==
  note: To avoid having the first point at (x,y) = (0,0)
      | due to the wah the enable subsystem works
  note: Recalculation of the trajectory + flatness:
      | Done on initialization and when obstacle appears
  note: Current reference point
  blending_factor : Inport
  Constant : Constant  Value=r
  Constant1 : Constant  Value=t_values
  Constant2 : Constant  Value=d
  Constant3 : Constant  Value=T
  Constant6 : Constant  Value=initial_position
  Data Store Read : DataStoreRead  DataStoreName=trajectory_x  IndexOptions=Index vector (dialog)  Indices=1  OutputSizes=1
  Data Store Read1 : DataStoreRead  DataStoreName=trajectory_y  IndexOptions=Index vector (dialog)  Indices=1  OutputSizes=1
  Data Store Read2 : DataStoreRead  DataStoreName=recalculate  IndexOptions=Index vector (dialog)  Indices=1  OutputSizes=1
  Data Store Write : DataStoreWrite  DataStoreName=recalculate  IndexOptions=Index vector (dialog)  Indices=1  OutputSizes=1
  Data Store Write1 : DataStoreWrite  DataStoreName=recalculate_obs  IndexOptions=Index vector (dialog)  Indices=1  OutputSizes=1
  Data Store Write2 : DataStoreWrite  DataStoreName=trajectory_x  IndexOptions=Index vector (dialog)  Indices=1  OutputSizes=1
  Data Store Write3 : DataStoreWrite  DataStoreName=trajectory_y  IndexOptions=Index vector (dialog)  Indices=1  OutputSizes=1
  Data Store Write4 : DataStoreWrite  DataStoreName=v_d_array  IndexOptions=Index vector (dialog)  Indices=1  OutputSizes=1
  Data Store Write5 : DataStoreWrite  DataStoreName=omega_d_array  IndexOptions=Index vector (dialog)  Indices=1  OutputSizes=1
  Data Store Write6 : DataStoreWrite  DataStoreName=theta_d_array  IndexOptions=Index vector (dialog)  Indices=1  OutputSizes=1
  MATLAB Function : MATLAB Function  TreatAsAtomicUnit=on
  NOT : Logic  Operator=NOT  IconShape=distinctive  AllPortsSameDT=off  OutDataTypeStr=boolean
  OR : Logic  Operator=OR  IconShape=distinctive  AllPortsSameDT=off  OutDataTypeStr=boolean
  Obstacle Detection : Subsystem
  Subsystem1 : Subsystem
  Subsystem3 : Subsystem
  x_d : Outport
  y_d : Outport  Port=2
  v_d : Outport  Port=3
  omega_d : Outport  Port=4
  theta_d : Outport  Port=5
  wires:
  Constant/1 -> Subsystem1/3(r)
  Constant1/1 -> Subsystem1/4(t_values)
  NOT/1 -> Subsystem3/Enable
  Constant2/1 -> Subsystem1/6(d)
  Data Store Read2/1 -> OR/2
  OR/1 -> NOT/1, Subsystem1/Enable  "recalculating_trajectory"
  Subsystem1/7(theta_d_array) -> Data Store Write6/1
  Subsystem1/6(omega_d_array) -> Data Store Write5/1
  Subsystem1/5(v_d_array) -> Data Store Write4/1
  Subsystem1/4(trajectory_y) -> Data Store Write3/1
  Subsystem1/3(trajectory_x) -> Data Store Write2/1
  Subsystem1/1(recalculate) -> Data Store Write/1
  Constant3/1 -> Subsystem1/5(T)
  Subsystem3/1(x_d) -> MATLAB Function/2(x1)
  MATLAB Function/1(x) -> x_d/1
  Subsystem3/2(y_d) -> MATLAB Function/3(y1)
  MATLAB Function/2(y) -> y_d/1
  MATLAB Function/3(v) -> v_d/1
  Subsystem3/3(v_d) -> MATLAB Function/4(v1)
  Subsystem3/4(omega_d) -> MATLAB Function/5(omega1)
  Subsystem3/5(theta_d) -> MATLAB Function/6(theta1)
  MATLAB Function/4(omega) -> omega_d/1
  MATLAB Function/5(theta) -> theta_d/1
  Constant6/1 -> MATLAB Function/1(initial_position)
  Subsystem3/6(new_i) -> MATLAB Function/7(i)
  Subsystem1/2(recalculate_obs) -> Data Store Write1/1
  blending_factor/1 -> Subsystem1/7(blending)
  Data Store Read/1 -> Subsystem1/8(old_traj_x)
  Data Store Read1/1 -> Subsystem1/9(old_traj_y)
  Obstacle Detection/1(recalc_obs) -> OR/1, Subsystem1/1(recalc_obs)
  [x] -> Obstacle Detection/1(Input)
  [y] -> Obstacle Detection/2(Input1)
  [theta] -> Obstacle Detection/3(Input2)
  [x1] -> Subsystem1/10(xd)
  [y1] -> Subsystem1/11(yd)
  [theta11] -> Subsystem1/2(theta)

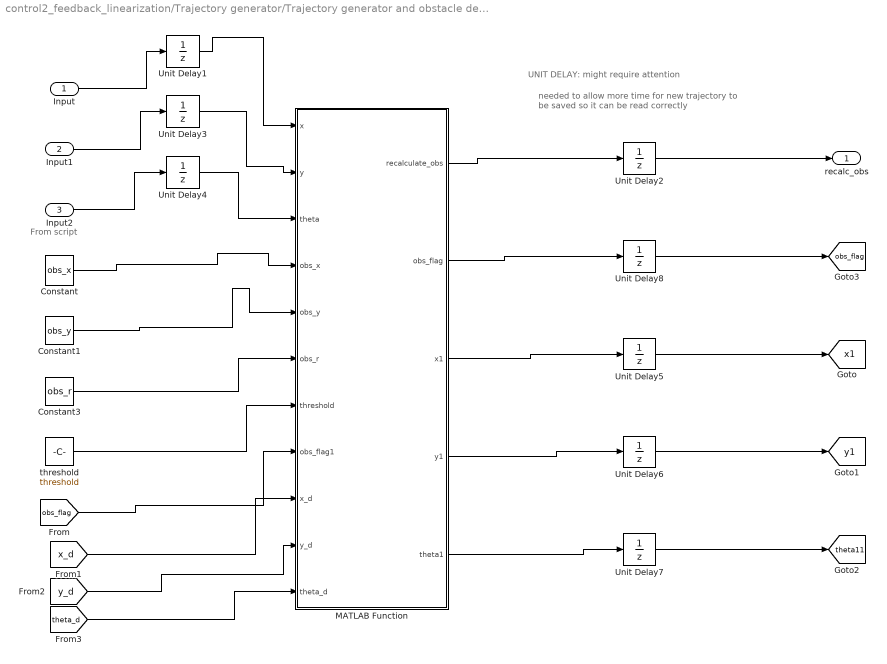
== system control2_feedback_linearization/Trajectory generator/Trajectory generator and obstacle detection/Obstacle Detection ==
  note: UNIT DELAY: might require attention
  note: needed to allow more time for new trajectory to be saved
      | so it can be read correctly
  note: From script
  Input : Inport
  Input1 : Inport  Port=2
  Input2 : Inport  Port=3
  Constant : Constant  Value=obs_x
  Constant1 : Constant  Value=obs_y
  Constant3 : Constant  Value=obs_r
  MATLAB Function : MATLAB Function  TreatAsAtomicUnit=on
  Unit Delay{1..8} (8 alike) : UnitDelay  SampleTime=0.001  HasFrameUpgradeWarning=on
  threshold : Constant  Value=threshold
  recalc_obs : Outport
  tag scope: obs_flag=global, theta11=global, x1=global, y1=global
  wires:
  Constant/1 -> MATLAB Function/4(obs_x)
  Constant1/1 -> MATLAB Function/5(obs_y)
  Constant3/1 -> MATLAB Function/6(obs_r)
  threshold/1 -> MATLAB Function/7(threshold)
  [obs_flag] -> MATLAB Function/8(obs_flag1)
  MATLAB Function/2(obs_flag) -> Unit Delay8/1
  MATLAB Function/1(recalculate_obs) -> Unit Delay2/1
  Input/1 -> Unit Delay1/1
  Input1/1 -> Unit Delay3/1
  Unit Delay2/1 -> recalc_obs/1
  Unit Delay1/1 -> MATLAB Function/1(x)
  Unit Delay3/1 -> MATLAB Function/2(y)
  Input2/1 -> Unit Delay4/1
  Unit Delay4/1 -> MATLAB Function/3(theta)
  MATLAB Function/3(x1) -> Unit Delay5/1
  Unit Delay5/1 -> [x1]
  MATLAB Function/4(y1) -> Unit Delay6/1
  Unit Delay6/1 -> [y1]
  MATLAB Function/5(theta1) -> Unit Delay7/1
  Unit Delay7/1 -> [theta11]
  Unit Delay8/1 -> [obs_flag]
  [x_d] -> MATLAB Function/9(x_d)
  [y_d] -> MATLAB Function/10(y_d)
  [theta_d] -> MATLAB Function/11(theta_d)

== system control2_feedback_linearization/Trajectory generator/Trajectory generator and obstacle detection/Subsystem1 ==
  recalc_obs : Inport
  theta : Inport  Port=2
  r : Inport  Port=3
  t_values : Inport  Port=4
  T : Inport  Port=5
  d : Inport  Port=6
  blending : Inport  Port=7
  old_traj_x : Inport  Port=8
  old_traj_y : Inport  Port=9
  xd : Inport  Port=10
  yd : Inport  Port=11
  Enable : EnablePort
  Whole trajectory calculation + flatness : MATLAB Function  TreatAsAtomicUnit=on
  recalculate : Outport
  recalculate_obs : Outport  Port=2
  trajectory_x : Outport  Port=3
  trajectory_y : Outport  Port=4
  v_d_array : Outport  Port=5
  omega_d_array : Outport  Port=6
  theta_d_array : Outport  Port=7
  wires:
  r/1 -> Whole trajectory calculation + flatness/1(r)
  Whole trajectory calculation + flatness/6(recalculate) -> recalculate/1
  t_values/1 -> Whole trajectory calculation + flatness/2(t_values)
  recalc_obs/1 -> Whole trajectory calculation + flatness/4(recalculate_obs)
  theta/1 -> Whole trajectory calculation + flatness/7(theta11)
  d/1 -> Whole trajectory calculation + flatness/5(d)
  Whole trajectory calculation + flatness/1(trajectory_x) -> trajectory_x/1
  Whole trajectory calculation + flatness/2(trajectory_y) -> trajectory_y/1
  Whole trajectory calculation + flatness/3(v_d_array) -> v_d_array/1
  Whole trajectory calculation + flatness/4(omega_d_array) -> omega_d_array/1
  Whole trajectory calculation + flatness/5(theta_d_array) -> theta_d_array/1
  T/1 -> Whole trajectory calculation + flatness/3(T)
  Whole trajectory calculation + flatness/7(recalculate_obs1) -> recalculate_obs/1
  blending/1 -> Whole trajectory calculation + flatness/6(blending)
  old_traj_x/1 -> Whole trajectory calculation + flatness/10(old_trajectory_x)
  old_traj_y/1 -> Whole trajectory calculation + flatness/11(old_trajectory_y)
  xd/1 -> Whole trajectory calculation + flatness/8(xd)
  yd/1 -> Whole trajectory calculation + flatness/9(yd)

== system control2_feedback_linearization/Trajectory generator/Trajectory generator and obstacle detection/Subsystem3 ==
  Enable : EnablePort
  Clock1 : Clock
  Constant3 : Constant  Value=t_values
  Data Store Read : DataStoreRead  DataStoreName=iteration  IndexOptions=Index vector (dialog)  Indices=1  OutputSizes=1
  Data Store Read11 : DataStoreRead  DataStoreName=trajectory_x  IndexOptions=Index vector (dialog)  Indices=1  OutputSizes=1
  Data Store Read12 : DataStoreRead  DataStoreName=trajectory_y  IndexOptions=Index vector (dialog)  Indices=1  OutputSizes=1
  Data Store Read13 : DataStoreRead  DataStoreName=v_d_array  IndexOptions=Index vector (dialog)  Indices=1  OutputSizes=1
  Data Store Read14 : DataStoreRead  DataStoreName=omega_d_array  IndexOptions=Index vector (dialog)  Indices=1  OutputSizes=1
  Data Store Read15 : DataStoreRead  DataStoreName=theta_d_array  IndexOptions=Index vector (dialog)  Indices=1  OutputSizes=1
  Data Store Write : DataStoreWrite  DataStoreName=iteration  IndexOptions=Index vector (dialog)  Indices=1  OutputSizes=1
  Triggered Subsystem : Subsystem  TreatAsAtomicUnit=on
  x_d : Outport
  y_d : Outport  Port=2
  v_d : Outport  Port=3
  omega_d : Outport  Port=4
  theta_d : Outport  Port=5
  new_i : Outport  Port=6
  wires:
  Triggered Subsystem/3(v_d) -> v_d/1
  Triggered Subsystem/1(x_d) -> x_d/1
  Triggered Subsystem/2(y_d) -> y_d/1
  Data Store Read12/1 -> Triggered Subsystem/4(trajectory_y)
  Triggered Subsystem/4(omega_d) -> omega_d/1
  Data Store Read15/1 -> Triggered Subsystem/7(theta_d_array)
  Data Store Read14/1 -> Triggered Subsystem/6(omega_d_array)
  Data Store Read11/1 -> Triggered Subsystem/3(trajectory_x)
  Data Store Read13/1 -> Triggered Subsystem/5(v_d_array)
  Triggered Subsystem/5(theta_d) -> theta_d/1
  Clock1/1 -> Triggered Subsystem/1(t)
  Constant3/1 -> Triggered Subsystem/2(t_values)
  Data Store Read/1 -> Triggered Subsystem/8(Input)
  Triggered Subsystem/6(new_i) -> Data Store Write/1, new_i/1

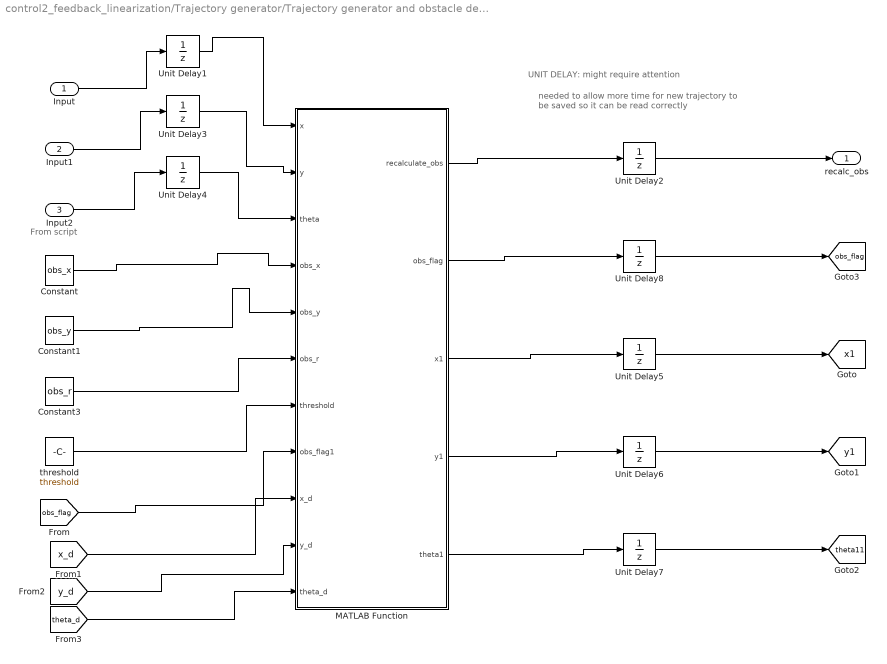
== system control2_feedback_linearization/Trajectory generator/Trajectory generator and obstacle detection1/Obstacle Detection ==
  note: UNIT DELAY: might require attention
  note: needed to allow more time for new trajectory to be saved
      | so it can be read correctly
  note: From script
  Input : Inport
  Input1 : Inport  Port=2
  Input2 : Inport  Port=3
  Constant : Constant  Value=obs_x
  Constant1 : Constant  Value=obs_y
  Constant3 : Constant  Value=obs_r
  MATLAB Function : MATLAB Function  TreatAsAtomicUnit=on
  Unit Delay{1..8} (8 alike) : UnitDelay  SampleTime=0.001  HasFrameUpgradeWarning=on
  threshold : Constant  Value=threshold
  recalc_obs : Outport
  tag scope: obs_flag=global, theta11=global, x1=global, y1=global
  wires:
  Constant/1 -> MATLAB Function/4(obs_x)
  Constant1/1 -> MATLAB Function/5(obs_y)
  Constant3/1 -> MATLAB Function/6(obs_r)
  threshold/1 -> MATLAB Function/7(threshold)
  [obs_flag] -> MATLAB Function/8(obs_flag1)
  MATLAB Function/2(obs_flag) -> Unit Delay8/1
  MATLAB Function/1(recalculate_obs) -> Unit Delay2/1
  Input/1 -> Unit Delay1/1
  Input1/1 -> Unit Delay3/1
  Unit Delay2/1 -> recalc_obs/1
  Unit Delay1/1 -> MATLAB Function/1(x)
  Unit Delay3/1 -> MATLAB Function/2(y)
  Input2/1 -> Unit Delay4/1
  Unit Delay4/1 -> MATLAB Function/3(theta)
  MATLAB Function/3(x1) -> Unit Delay5/1
  Unit Delay5/1 -> [x1]
  MATLAB Function/4(y1) -> Unit Delay6/1
  Unit Delay6/1 -> [y1]
  MATLAB Function/5(theta1) -> Unit Delay7/1
  Unit Delay7/1 -> [theta11]
  Unit Delay8/1 -> [obs_flag]
  [x_d] -> MATLAB Function/9(x_d)
  [y_d] -> MATLAB Function/10(y_d)
  [theta_d] -> MATLAB Function/11(theta_d)

== system control2_feedback_linearization/Trajectory generator/Trajectory generator and obstacle detection1/Subsystem1 ==
  recalc_obs : Inport
  theta : Inport  Port=2
  r : Inport  Port=3
  t_values : Inport  Port=4
  T : Inport  Port=5
  d : Inport  Port=6
  blending : Inport  Port=7
  old_traj_x : Inport  Port=8
  old_traj_y : Inport  Port=9
  xd : Inport  Port=10
  yd : Inport  Port=11
  Enable : EnablePort
  Whole trajectory calculation + flatness : MATLAB Function  TreatAsAtomicUnit=on
  recalculate : Outport
  recalculate_obs : Outport  Port=2
  trajectory_x : Outport  Port=3
  trajectory_y : Outport  Port=4
  v_d_array : Outport  Port=5
  omega_d_array : Outport  Port=6
  theta_d_array : Outport  Port=7
  wires:
  r/1 -> Whole trajectory calculation + flatness/1(r)
  Whole trajectory calculation + flatness/6(recalculate) -> recalculate/1
  t_values/1 -> Whole trajectory calculation + flatness/2(t_values)
  recalc_obs/1 -> Whole trajectory calculation + flatness/4(recalculate_obs)
  theta/1 -> Whole trajectory calculation + flatness/7(theta11)
  d/1 -> Whole trajectory calculation + flatness/5(d)
  Whole trajectory calculation + flatness/1(trajectory_x) -> trajectory_x/1
  Whole trajectory calculation + flatness/2(trajectory_y) -> trajectory_y/1
  Whole trajectory calculation + flatness/3(v_d_array) -> v_d_array/1
  Whole trajectory calculation + flatness/4(omega_d_array) -> omega_d_array/1
  Whole trajectory calculation + flatness/5(theta_d_array) -> theta_d_array/1
  T/1 -> Whole trajectory calculation + flatness/3(T)
  Whole trajectory calculation + flatness/7(recalculate_obs1) -> recalculate_obs/1
  blending/1 -> Whole trajectory calculation + flatness/6(blending)
  old_traj_x/1 -> Whole trajectory calculation + flatness/10(old_trajectory_x)
  old_traj_y/1 -> Whole trajectory calculation + flatness/11(old_trajectory_y)
  xd/1 -> Whole trajectory calculation + flatness/8(xd)
  yd/1 -> Whole trajectory calculation + flatness/9(yd)

== system control2_feedback_linearization/Trajectory generator/Trajectory generator and obstacle detection1/Subsystem3 ==
  Enable : EnablePort
  Clock1 : Clock
  Constant3 : Constant  Value=t_values
  Data Store Read : DataStoreRead  DataStoreName=iteration  IndexOptions=Index vector (dialog)  Indices=1  OutputSizes=1
  Data Store Read11 : DataStoreRead  DataStoreName=trajectory_x  IndexOptions=Index vector (dialog)  Indices=1  OutputSizes=1
  Data Store Read12 : DataStoreRead  DataStoreName=trajectory_y  IndexOptions=Index vector (dialog)  Indices=1  OutputSizes=1
  Data Store Read13 : DataStoreRead  DataStoreName=v_d_array  IndexOptions=Index vector (dialog)  Indices=1  OutputSizes=1
  Data Store Read14 : DataStoreRead  DataStoreName=omega_d_array  IndexOptions=Index vector (dialog)  Indices=1  OutputSizes=1
  Data Store Read15 : DataStoreRead  DataStoreName=theta_d_array  IndexOptions=Index vector (dialog)  Indices=1  OutputSizes=1
  Data Store Write : DataStoreWrite  DataStoreName=iteration  IndexOptions=Index vector (dialog)  Indices=1  OutputSizes=1
  Triggered Subsystem : Subsystem  TreatAsAtomicUnit=on
  x_d : Outport
  y_d : Outport  Port=2
  v_d : Outport  Port=3
  omega_d : Outport  Port=4
  theta_d : Outport  Port=5
  new_i : Outport  Port=6
  wires:
  Triggered Subsystem/3(v_d) -> v_d/1
  Triggered Subsystem/1(x_d) -> x_d/1
  Triggered Subsystem/2(y_d) -> y_d/1
  Data Store Read12/1 -> Triggered Subsystem/4(trajectory_y)
  Triggered Subsystem/4(omega_d) -> omega_d/1
  Data Store Read15/1 -> Triggered Subsystem/7(theta_d_array)
  Data Store Read14/1 -> Triggered Subsystem/6(omega_d_array)
  Data Store Read11/1 -> Triggered Subsystem/3(trajectory_x)
  Data Store Read13/1 -> Triggered Subsystem/5(v_d_array)
  Triggered Subsystem/5(theta_d) -> theta_d/1
  Clock1/1 -> Triggered Subsystem/1(t)
  Constant3/1 -> Triggered Subsystem/2(t_values)
  Data Store Read/1 -> Triggered Subsystem/8(Input)
  Triggered Subsystem/6(new_i) -> Data Store Write/1, new_i/1

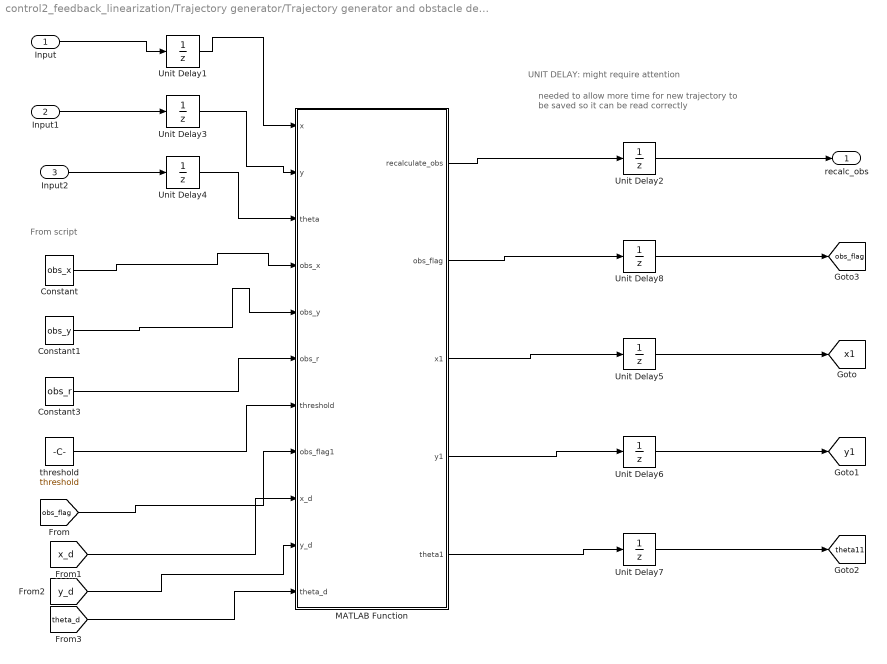
== system control2_feedback_linearization/Trajectory generator/Trajectory generator and obstacle detection2/Obstacle Detection ==
  note: UNIT DELAY: might require attention
  note: needed to allow more time for new trajectory to be saved
      | so it can be read correctly
  note: From script
  Input : Inport
  Input1 : Inport  Port=2
  Input2 : Inport  Port=3
  Constant : Constant  Value=obs_x
  Constant1 : Constant  Value=obs_y
  Constant3 : Constant  Value=obs_r
  MATLAB Function : MATLAB Function  TreatAsAtomicUnit=on
  Unit Delay{1..8} (8 alike) : UnitDelay  SampleTime=0.001  HasFrameUpgradeWarning=on
  threshold : Constant  Value=threshold
  recalc_obs : Outport
  tag scope: obs_flag=global, theta11=global, x1=global, y1=global
  wires:
  Constant/1 -> MATLAB Function/4(obs_x)
  Constant1/1 -> MATLAB Function/5(obs_y)
  Constant3/1 -> MATLAB Function/6(obs_r)
  threshold/1 -> MATLAB Function/7(threshold)
  [obs_flag] -> MATLAB Function/8(obs_flag1)
  MATLAB Function/2(obs_flag) -> Unit Delay8/1
  MATLAB Function/1(recalculate_obs) -> Unit Delay2/1
  Input/1 -> Unit Delay1/1
  Input1/1 -> Unit Delay3/1
  Unit Delay2/1 -> recalc_obs/1
  Unit Delay1/1 -> MATLAB Function/1(x)
  Unit Delay3/1 -> MATLAB Function/2(y)
  Input2/1 -> Unit Delay4/1
  Unit Delay4/1 -> MATLAB Function/3(theta)
  MATLAB Function/3(x1) -> Unit Delay5/1
  Unit Delay5/1 -> [x1]
  MATLAB Function/4(y1) -> Unit Delay6/1
  Unit Delay6/1 -> [y1]
  MATLAB Function/5(theta1) -> Unit Delay7/1
  Unit Delay7/1 -> [theta11]
  Unit Delay8/1 -> [obs_flag]
  [x_d] -> MATLAB Function/9(x_d)
  [y_d] -> MATLAB Function/10(y_d)
  [theta_d] -> MATLAB Function/11(theta_d)

== system control2_feedback_linearization/Trajectory generator/Trajectory generator and obstacle detection2/Subsystem1 ==
  recalc_obs : Inport
  theta : Inport  Port=2
  r : Inport  Port=3
  t_values : Inport  Port=4
  T : Inport  Port=5
  d : Inport  Port=6
  blending : Inport  Port=7
  old_traj_x : Inport  Port=8
  old_traj_y : Inport  Port=9
  xd : Inport  Port=10
  yd : Inport  Port=11
  Enable : EnablePort
  Whole trajectory calculation + flatness : MATLAB Function  TreatAsAtomicUnit=on
  recalculate : Outport
  recalculate_obs : Outport  Port=2
  trajectory_x : Outport  Port=3
  trajectory_y : Outport  Port=4
  v_d_array : Outport  Port=5
  omega_d_array : Outport  Port=6
  theta_d_array : Outport  Port=7
  wires:
  r/1 -> Whole trajectory calculation + flatness/1(r)
  Whole trajectory calculation + flatness/6(recalculate) -> recalculate/1
  t_values/1 -> Whole trajectory calculation + flatness/2(t_values)
  recalc_obs/1 -> Whole trajectory calculation + flatness/4(recalculate_obs)
  theta/1 -> Whole trajectory calculation + flatness/7(theta11)
  d/1 -> Whole trajectory calculation + flatness/5(d)
  Whole trajectory calculation + flatness/1(trajectory_x) -> trajectory_x/1
  Whole trajectory calculation + flatness/2(trajectory_y) -> trajectory_y/1
  Whole trajectory calculation + flatness/3(v_d_array) -> v_d_array/1
  Whole trajectory calculation + flatness/4(omega_d_array) -> omega_d_array/1
  Whole trajectory calculation + flatness/5(theta_d_array) -> theta_d_array/1
  T/1 -> Whole trajectory calculation + flatness/3(T)
  Whole trajectory calculation + flatness/7(recalculate_obs1) -> recalculate_obs/1
  blending/1 -> Whole trajectory calculation + flatness/6(blending)
  old_traj_x/1 -> Whole trajectory calculation + flatness/10(old_trajectory_x)
  old_traj_y/1 -> Whole trajectory calculation + flatness/11(old_trajectory_y)
  xd/1 -> Whole trajectory calculation + flatness/8(xd)
  yd/1 -> Whole trajectory calculation + flatness/9(yd)
